simulink model "pidsimu_teacher_fig1"  (R2022a)
settings: Solver=ode45  StartTime=0.0  StopTime=60  MaxStep=1  MinStep=0.001  RelTol=1e-2  EnableMultiTasking=on
settings Model: Creator=slack  LastModifiedBy=slack
settings SolverCC: InitialStep=0.01
settings DataIOCC: LimitDataPoints=on  SaveFormat=Array  SignalLoggingSaveFormat=ModelDataLogs  ReturnWorkspaceOutputs=off  SignalLoggingName=sigsOut  Refine=3
settings OptimizationCC: OptimizeBlockIOStorage=off  BufferReuse=off  ExpressionFolding=off  LocalBlockOutputs=off  InitFltsAndDblsToZero=on  LifeSpan=inf
settings DebuggingCC: SaveWithParameterizedLinksMsg=none  UnderspecifiedInitializationDetection=Classic  MergeDetectMultiDrivingBlocksExec=none  SignalResolutionControl=TryResolveAllWithWarning  MultiTaskDSMMsg=warning  MultiTaskCondExecSysMsg=none  UnconnectedInputMsg=warning  UnconnectedOutputMsg=warning  UnconnectedLineMsg=warning  SFUnexpectedBacktrackingDiag=warning  SFNoUnconditionalDefaultTransitionDiag=warning  SFExecutionAtInitializationDiag=none  SFMachineParentedDataDiag=warning  ArithmeticOperatorsInVariantConditions=warning
settings HardwareCC: ProdBitPerPointer=32  ProdBitPerSizeT=32  ProdBitPerPtrDiffT=32  ProdLargestAtomicFloat=None  ProdIntDivRoundTo=Undefined  ProdEndianess=Unspecified  ProdWordSize=32  ProdHWDeviceType=32-bit Generic  TargetUnknown=on
settings ModelReferenceCC: PropagateSignalLabelsOutOfModel=off
settings CodeAppCC: StateflowObjectComments=on
settings GRTTargetCC: TargetFcnLib=ansi_tfl_tmw.mat  TargetLangStandard=C89/C90 (ANSI)  CombineOutputUpdateFcns=off  GRTInterface=on
settings ConfigComp: CovMetricSettings=dw  CovSaveCumulativeToWorkspaceVar=on  CovSaveSingleToWorkspaceVar=on

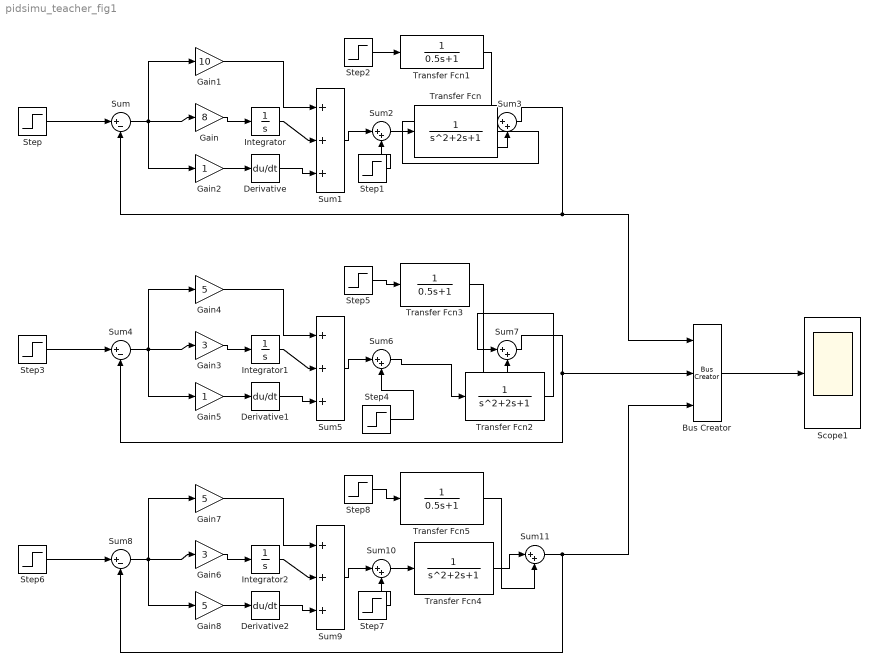
== system pidsimu_teacher_fig1 ==
  Bus Creator : BusCreator  Inputs=3
  Derivative : Derivative
  Derivative1 : Derivative
  Derivative2 : Derivative
  Gain : Gain  Gain=8  SaturateOnIntegerOverflow=on  OutDataTypeStr=Inherit: Same as input  ParamDataTypeStr=Inherit: Same as input
  Gain1 : Gain  Gain=10  SaturateOnIntegerOverflow=on  OutDataTypeStr=Inherit: Same as input  ParamDataTypeStr=Inherit: Same as input
  Gain2 : Gain  SaturateOnIntegerOverflow=on  OutDataTypeStr=Inherit: Same as input  ParamDataTypeStr=Inherit: Same as input
  Gain3 : Gain  Gain=3  SaturateOnIntegerOverflow=on  OutDataTypeStr=Inherit: Same as input  ParamDataTypeStr=Inherit: Same as input
  Gain4 : Gain  Gain=5  SaturateOnIntegerOverflow=on  OutDataTypeStr=Inherit: Same as input  ParamDataTypeStr=Inherit: Same as input
  Gain5 : Gain  SaturateOnIntegerOverflow=on  OutDataTypeStr=Inherit: Same as input  ParamDataTypeStr=Inherit: Same as input
  Gain6 : Gain  Gain=3  SaturateOnIntegerOverflow=on  OutDataTypeStr=Inherit: Same as input  ParamDataTypeStr=Inherit: Same as input
  Gain7 : Gain  Gain=5  SaturateOnIntegerOverflow=on  OutDataTypeStr=Inherit: Same as input  ParamDataTypeStr=Inherit: Same as input
  Gain8 : Gain  Gain=5  SaturateOnIntegerOverflow=on  OutDataTypeStr=Inherit: Same as input  ParamDataTypeStr=Inherit: Same as input
  Integrator : Integrator
  Integrator1 : Integrator
  Integrator2 : Integrator
  Scope1 : Scope
  Step : Step  Time=0  SampleTime=0.1
  Step1 : Step  Time=20  SampleTime=0.1
  Step2 : Step  Time=40  SampleTime=0.1
  Step3 : Step  Time=0  SampleTime=0.1
  Step4 : Step  Time=20  SampleTime=0.1
  Step5 : Step  Time=40  SampleTime=0.1
  Step6 : Step  Time=0  SampleTime=0.1
  Step7 : Step  Time=20  SampleTime=0.1
  Step8 : Step  Time=40  SampleTime=0.1
  Sum : Sum  Inputs=|+-  SaturateOnIntegerOverflow=on
  Sum1 : Sum  Inputs=|+++  SaturateOnIntegerOverflow=on
  Sum{2..3,6..7,10..11} (6 alike) : Sum  Inputs=|++  SaturateOnIntegerOverflow=on
  Sum4 : Sum  Inputs=|+-  SaturateOnIntegerOverflow=on
  Sum5 : Sum  Inputs=|+++  SaturateOnIntegerOverflow=on
  Sum8 : Sum  Inputs=|+-  SaturateOnIntegerOverflow=on
  Sum9 : Sum  Inputs=|+++  SaturateOnIntegerOverflow=on
  Transfer Fcn : TransferFcn  Numerator=[1 ]
  Transfer Fcn1 : TransferFcn  Numerator=[1 ]  Denominator=[ 0.5 1]
  Transfer Fcn2 : TransferFcn  Numerator=[1 ]
  Transfer Fcn3 : TransferFcn  Numerator=[1 ]  Denominator=[ 0.5 1]
  Transfer Fcn4 : TransferFcn  Numerator=[1 ]
  Transfer Fcn5 : TransferFcn  Numerator=[1 ]  Denominator=[ 0.5 1]
  wires:
  Step/1 -> Sum/1
  Sum/1 -> Gain/1, Gain2/1, Gain1/1
  Gain1/1 -> Sum1/1
  Gain/1 -> Integrator/1
  Integrator/1 -> Sum1/2
  Gain2/1 -> Derivative/1
  Derivative/1 -> Sum1/3
  Sum1/1 -> Sum2/1
  Sum2/1 -> Transfer Fcn/1
  Step1/1 -> Sum2/2
  Step2/1 -> Transfer Fcn1/1
  Transfer Fcn/1 -> Sum3/1
  Sum3/1 -> Bus Creator/1, Sum/2
  Transfer Fcn1/1 -> Sum3/2
  Step3/1 -> Sum4/1
  Sum4/1 -> Gain3/1, Gain5/1, Gain4/1
  Gain4/1 -> Sum5/1
  Gain3/1 -> Integrator1/1
  Integrator1/1 -> Sum5/2
  Gain5/1 -> Derivative1/1
  Derivative1/1 -> Sum5/3
  Sum5/1 -> Sum6/1
  Sum6/1 -> Transfer Fcn2/1
  Step4/1 -> Sum6/2
  Step5/1 -> Transfer Fcn3/1
  Transfer Fcn2/1 -> Sum7/1
  Sum7/1 -> Sum4/2, Bus Creator/2
  Transfer Fcn3/1 -> Sum7/2
  Step6/1 -> Sum8/1
  Sum8/1 -> Gain6/1, Gain8/1, Gain7/1
  Gain7/1 -> Sum9/1
  Gain6/1 -> Integrator2/1
  Integrator2/1 -> Sum9/2
  Gain8/1 -> Derivative2/1
  Derivative2/1 -> Sum9/3
  Sum9/1 -> Sum10/1
  Sum10/1 -> Transfer Fcn4/1
  Step7/1 -> Sum10/2
  Step8/1 -> Transfer Fcn5/1
  Transfer Fcn4/1 -> Sum11/1
  Sum11/1 -> Bus Creator/3, Sum8/2
  Transfer Fcn5/1 -> Sum11/2
  Bus Creator/1 -> Scope1/1
